simulink model "test_4"  (R2022b)
settings: Solver=ode1  StartTime=0.0  StopTime=.5  FixedStep=.01  RelTol=1e-3  AbsTol=1e-3
values from neighbouring files (symbols this model uses):
  Ts = .05    (= 0.05)    [RunMeFirst.m]    (also in linsys1.m = 0.1)
settings Model: Creator=Sajjad  LastModifiedBy=hp_desktop
settings SolverCC: AutoScaleAbsTol=off
settings OptimizationCC: BlockReduction=off  OptimizeBlockIOStorage=off

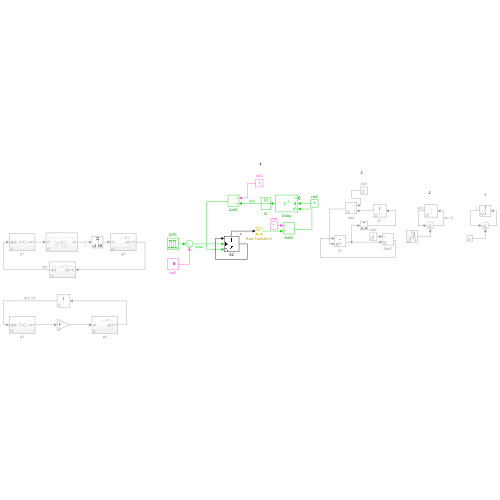
[thumbnail: Simulink's stored preview of the top-level diagram]
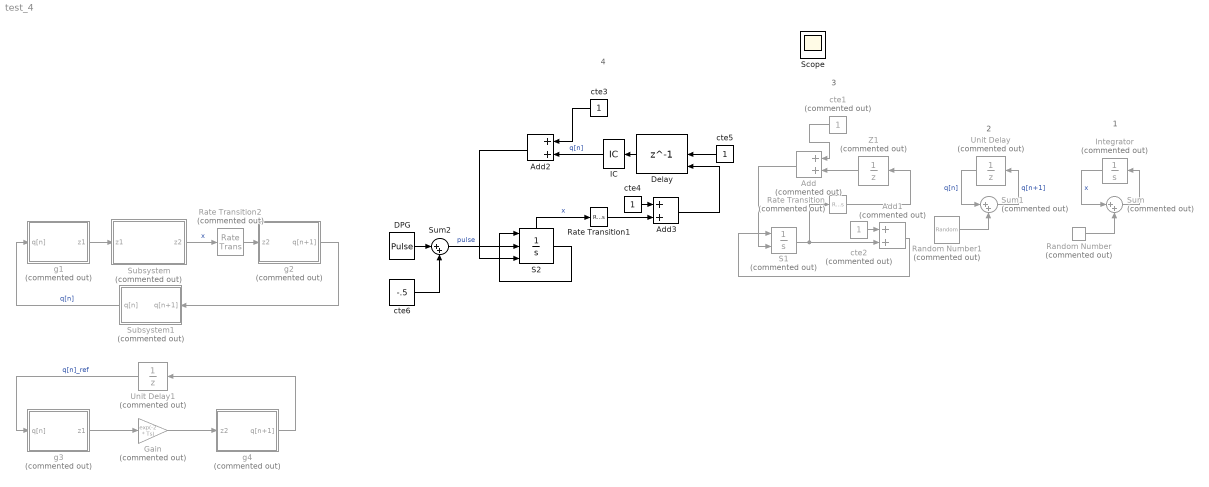
== system test_4 ==
  note: 2
  note: 1
  note: 3
  note: 4
  Add : Sum  Commented=on
  Add1 : Sum  Commented=on
  Add2 : Sum
  Add3 : Sum
  DPG : DiscretePulseGenerator  SampleTime=.03
  Delay : Delay  DelayLength=1  InitialConditionSource=Input port  ExternalReset=Level hold  SampleTime=.03
      settings: InputPortMap=u0,r5,p4
  Gain : Gain  Commented=on  Gain=exp(-2 * Ts)
  IC : InitialCondition  Value=0
  Integrator : Integrator  Commented=on  InitialCondition=1e-2
  Random Number : RandomNumber  Commented=on  SampleTime=0.1
  Random Number1 : RandomNumber  Commented=on  SampleTime=0
  Rate Transition : RateTransition  Commented=on  OutPortSampleTime=.03
  Rate Transition1 : RateTransition  OutPortSampleTime=.03
  Rate Transition2 : RateTransition  Commented=on  OutPortSampleTime=Ts
  S1 : Integrator  Commented=on  InitialConditionSource=external
  S2 : Integrator  ExternalReset=either  InitialConditionSource=external  ShowStatePort=on
  Subsystem : Subsystem  Commented=on
  Subsystem1 : Subsystem  Commented=on
      settings: PortSchema="{\"entries\":[{\"content\":{\"sides\":[{\"content\":{\"connectorIds\":[\"Out1\"]},\"type\":\"ConnectorPlacement.EquallySpacedRectSide\",\"uuid\":\"8fc94844-539d-471e-85bc-9f62e8ce35eb\"},{\"content\":{\"connectorIds\":[\"In1\"],\"side\":\"RIGHT\"},\"type\":\"ConnectorPlacement.EquallySpacedRectSide\",\"uuid\":\"aaedb0e0-a2c0-49a6-bcd4-3aa071ce77d8\"},{\"content\":{\"connectorIds\":[],\"side\":\"TOP\"},\"type\":\"ConnectorPlacement.EquallySpacedRectSide\",\"uuid\":\"e03a8975-ad96-4a59-9323-f2b81042749a\"}]},\"type\":\"ConnectorPlacement.EquallySpacedConnector\",\"uuid\":\"625a6665-3eb5-44d0-a083-715313f2b0a8\"}],\"packageUris\":[\"http://schema.mathworks.com/mf0/Connector/R2020b\"],\"version\":\"1.0\"}"
  Sum : Sum  Commented=on  Inputs=|++
  Sum1 : Sum  Commented=on  Inputs=|++
  Sum2 : Sum  Inputs=|++
  Unit Delay : UnitDelay  Commented=on  SampleTime=-1  HasFrameUpgradeWarning=on
  Unit Delay1 : UnitDelay  Commented=on  SampleTime=Ts  HasFrameUpgradeWarning=on
  Z1 : UnitDelay  Commented=on  SampleTime=.03  HasFrameUpgradeWarning=on
  cte1 : Constant  Commented=on
  cte2 : Constant  Commented=on
  cte3 : Constant
  cte4 : Constant
  cte5 : Constant  SampleTime=.03
  cte6 : Constant  Value=-.5
  g1 : Subsystem  Commented=on
  g2 : Subsystem  Commented=on
  g3 : Subsystem  Commented=on
  g4 : Subsystem  Commented=on
  Scope : Scope
  wires:
  Integrator/1 -> Sum/1  "x"
  Sum/1 -> Integrator/1
  Random Number/1 -> Sum/2
  Random Number1/1 -> Sum1/2
  Unit Delay/1 -> Sum1/1  "q[n]"
  Sum1/1 -> Unit Delay/1  "q[n+1]"
  Add/1 -> S1/2
  cte1/1 -> Add/1
  Z1/1 -> Add/2
  cte2/1 -> Add1/1
  S1/1 -> Rate Transition/1, Add1/2
  Add1/1 -> S1/1
  Rate Transition/1 -> Z1/1
  Add2/1 -> S2/3
  Delay/1 -> IC/1
  cte4/1 -> Add3/1
  S2/1 -> S2/1
  cte3/1 -> Add2/1
  cte5/1 -> Delay/2
  Rate Transition1/1 -> Add3/2
  Add3/1 -> Delay/3
  IC/1 -> Add2/2  "q[n]"
  S2/State -> Rate Transition1/1  "x"
  DPG/1 -> Sum2/1
  cte6/1 -> Sum2/2
  Sum2/1 -> S2/2  "pulse"
  Subsystem/1(z2) -> Rate Transition2/1  "x"
  Rate Transition2/1 -> g2/1(z2)
  g2/1(q[n+1]) -> Subsystem1/1(q[n+1])
  Subsystem1/1(q[n]) -> g1/1(q[n])  "q[n]"
  g1/1(z1) -> Subsystem/1(z1)
  Unit Delay1/1 -> g3/1(q[n])  "q[n]_ref"
  g3/1(z1) -> Gain/1
  Gain/1 -> g4/1(z2)
  g4/1(q[n+1]) -> Unit Delay1/1

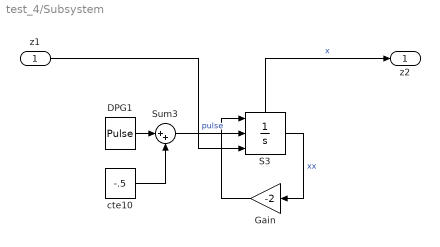
== system test_4/Subsystem ==
  z1 : Inport
  DPG1 : DiscretePulseGenerator  SampleTime=Ts
  Gain : Gain  Gain=-2
  S3 : Integrator  ExternalReset=either  InitialConditionSource=external  ShowStatePort=on
  Sum3 : Sum  Inputs=|++
  cte10 : Constant  Value=-.5
  z2 : Outport
  wires:
  Gain/1 -> S3/1
  cte10/1 -> Sum3/2
  Sum3/1 -> S3/2  "pulse"
  DPG1/1 -> Sum3/1
  S3/1 -> Gain/1  "xx"
  z1/1 -> S3/3
  S3/State -> z2/1  "x"

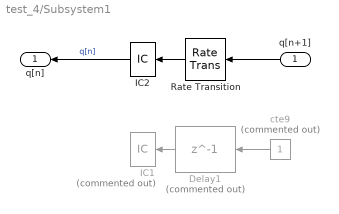
== system test_4/Subsystem1 ==
  q[n+1] : Inport
  Delay1 : Delay  Commented=on  DelayLength=1  InitialConditionSource=Input port  ExternalReset=Level hold  SampleTime=Ts
      settings: InputPortMap=u0,r5,p4
  IC1 : InitialCondition  Commented=on  Value=0
  IC2 : InitialCondition  Value=0
  Rate Transition : RateTransition  OutPortSampleTime=Ts
  cte9 : Constant  Commented=on  SampleTime=Ts
  q[n] : Outport
  wires:
  cte9/1 -> Delay1/2
  q[n+1]/1 -> Rate Transition/1
  Delay1/1 -> IC1/1
  Rate Transition/1 -> IC2/1
  IC2/1 -> q[n]/1  "q[n]"

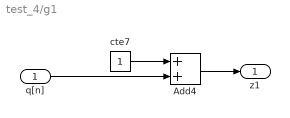
== system test_4/g1 ==
  q[n] : Inport
  Add4 : Sum
  cte7 : Constant
  z1 : Outport
  wires:
  cte7/1 -> Add4/1
  q[n]/1 -> Add4/2
  Add4/1 -> z1/1

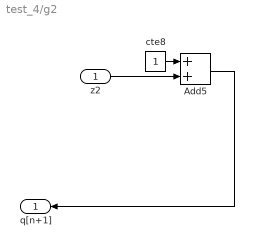
== system test_4/g2 ==
  z2 : Inport
  Add5 : Sum
  cte8 : Constant
  q[n+1] : Outport
  wires:
  z2/1 -> Add5/2
  cte8/1 -> Add5/1
  Add5/1 -> q[n+1]/1

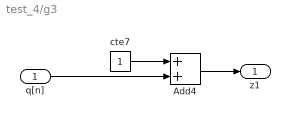
== system test_4/g3 ==
  q[n] : Inport
  Add4 : Sum
  cte7 : Constant
  z1 : Outport
  wires:
  Add4/1 -> z1/1
  q[n]/1 -> Add4/2
  cte7/1 -> Add4/1

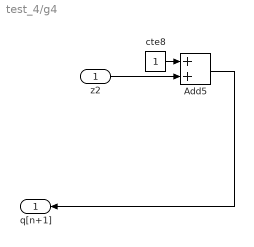
== system test_4/g4 ==
  z2 : Inport
  Add5 : Sum
  cte8 : Constant
  q[n+1] : Outport
  wires:
  Add5/1 -> q[n+1]/1
  cte8/1 -> Add5/1
  z2/1 -> Add5/2
